simulink model "controllers"  (Simulink 9.3)
settings: Solver=ode45  StartTime=0.0  StopTime=10.0  RelTol=1e-3  EnableMultiTasking=on
values from neighbouring files (symbols this model uses):
  C = [0  1]    [control_design.m]    (also in control_design_merged.m = [0 1])
  F = tf([K_pid*(Ti+Ti*Td*N) K_pid*(Ti*N+1) K_pid*N] , [Ti Ti*N 0])    [control_design.m]    (also in control_design_merged.m = K_pid * (1 + 1/(Ti*s) + Td*N*s/(s+N)))
  Gamma = sys2_prime.B    [control_design_merged.m]
  K = place(Phi' , C' , 5*pole(sys2_prime))    [control_design.m]    (also in control_design_merged.m = acker(Phi' , C' , discrete_poles_2).')
  L = acker(Phi , Gamma , pole(sys2_prime))    [control_design.m]    (also in control_design_merged.m = acker(Phi , Gamma , discrete_poles))
  lr = 1/(C * inv(eye(2) - Phi + Gamma*L) * Gamma)    [control_design.m]    (also in control_design_merged.m)
  Phi = sys2_prime.A    [control_design_merged.m]
  Ts = 4    [control_design.m]    (also in control_design_merged.m = 0.2)
undefined symbols (not defined in the file or in its folder): A_discretized, B_discretized, C_discretized, D_discretized
settings Model: Creator=umsonst  LastModifiedBy=RUOBING
settings DataIOCC: LimitDataPoints=on  SignalLoggingName=sigsOut
settings OptimizationCC: LifeSpan=auto
settings DebuggingCC: SaveWithParameterizedLinksMsg=none  SignalResolutionControl=TryResolveAllWithWarning  MultiTaskDSMMsg=warning  MultiTaskCondExecSysMsg=none  FcnCallInpInsideContextMsg=error  SFUnexpectedBacktrackingDiag=error  SFNoUnconditionalDefaultTransitionDiag=error  SFExecutionAtInitializationDiag=warning
settings HardwareCC: TargetUnknown=on

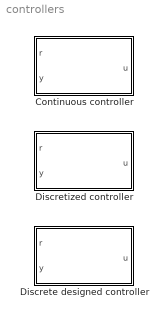
== system controllers ==
  Continuous controller : Subsystem
  Discrete designed controller : Subsystem
  Discretized controller : Subsystem

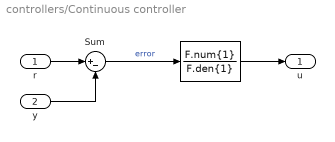
== system controllers/Continuous controller ==
  r : Inport
  y : Inport  Port=2
  " " : TransferFcn  Numerator=F.num{1}  Denominator=F.den{1}
  Sum : Sum  Inputs=|+-  SaturateOnIntegerOverflow=on
  u : Outport
  wires:
  Sum/1 -> " "/1  "error"
  y/1 -> Sum/2
  r/1 -> Sum/1
  " "/1 -> u/1

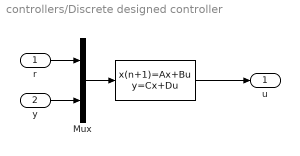
== system controllers/Discrete designed controller ==
  r : Inport
  y : Inport  Port=2
  "   " : DiscreteStateSpace  A=Phi-Gamma*L-K*C  B=[lr * Gamma K]  C=-L  D=[lr 0]  SampleTime=Ts
  Mux : Mux  Inputs=2
  u : Outport
  wires:
  r/1 -> Mux/1
  y/1 -> Mux/2
  Mux/1 -> "   "/1
  "   "/1 -> u/1

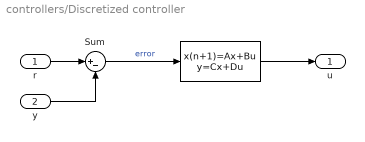
== system controllers/Discretized controller ==
  r : Inport
  y : Inport  Port=2
  " " : DiscreteStateSpace  A=A_discretized  B=B_discretized  C=C_discretized  D=D_discretized  SampleTime=Ts
  Sum : Sum  Inputs=|+-  SaturateOnIntegerOverflow=on
  u : Outport
  wires:
  Sum/1 -> " "/1  "error"
  y/1 -> Sum/2
  r/1 -> Sum/1
  " "/1 -> u/1
